simulink model "Linm_lin_1rob"  (Simulink 7.5)
settings: Solver=ode3  StartTime=0.0  StopTime=3  FixedStep=0.02  RelTol=1e-3
settings Model: Creator=FClaveau  LastModifiedBy=fclaveau
settings DebuggingCC: SaveWithParameterizedLinksMsg=none  MultiTaskCondExecSysMsg=none  StrictBusMsg=Warning
settings RTWCC: IncludeERTFirstTime=on

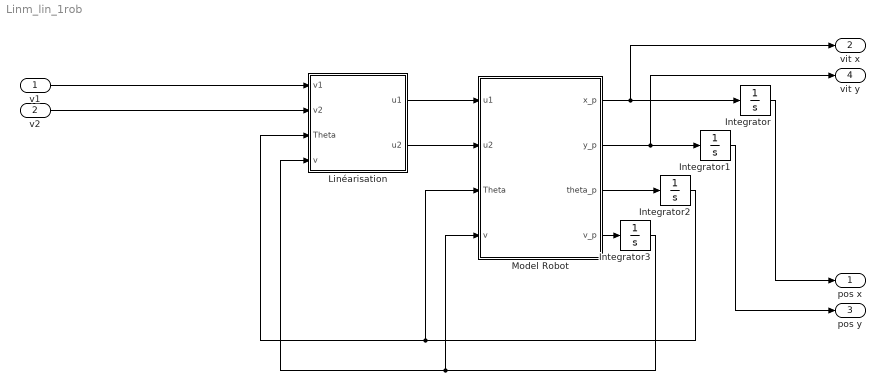
== system Linm_lin_1rob ==
  v1 : Inport
  v2 : Inport  Port=2
  Integrator : Integrator
  Integrator1 : Integrator
  Integrator2 : Integrator  InitialCondition=1
  Integrator3 : Integrator  InitialCondition=2
  Linéarisation : Subsystem
  Model Robot : Subsystem
  pos x : Outport
  vit x : Outport  Port=2
  pos y : Outport  Port=3
  vit y : Outport  Port=4
  wires:
  Model Robot/1(x_p) -> Integrator/1, vit x/1
  Model Robot/2(y_p) -> Integrator1/1, vit y/1
  Model Robot/3(theta_p) -> Integrator2/1
  Model Robot/4(v_p) -> Integrator3/1
  Integrator2/1 -> Model Robot/3(Theta), Linéarisation/3(Theta)
  Integrator3/1 -> Model Robot/4(v), Linéarisation/4(v)
  v2/1 -> Linéarisation/2(v2)
  Integrator/1 -> pos x/1
  Integrator1/1 -> pos y/1
  Linéarisation/1(u1) -> Model Robot/1(u1)
  Linéarisation/2(u2) -> Model Robot/2(u2)
  v1/1 -> Linéarisation/1(v1)

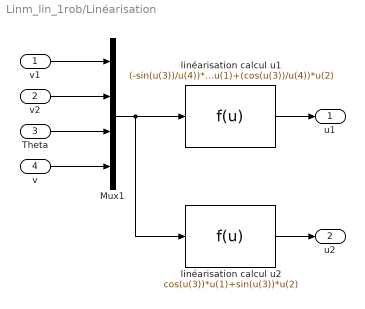
== system Linm_lin_1rob/Linéarisation ==
  v1 : Inport
  v2 : Inport  Port=2
  Theta : Inport  Port=3
  v : Inport  Port=4
  Mux1 : Mux
  linéarisation calcul u1 : Fcn  Expr=(-sin(u(3))/u(4))*u(1)+(cos(u(3))/u(4))*u(2)
  linéarisation calcul u2 : Fcn  Expr=cos(u(3))*u(1)+sin(u(3))*u(2)
  u1 : Outport
  u2 : Outport  Port=2
  wires:
  v1/1 -> Mux1/1
  v2/1 -> Mux1/2
  Theta/1 -> Mux1/3
  v/1 -> Mux1/4
  Mux1/1 -> linéarisation calcul u1/1, linéarisation calcul u2/1
  linéarisation calcul u2/1 -> u2/1
  linéarisation calcul u1/1 -> u1/1

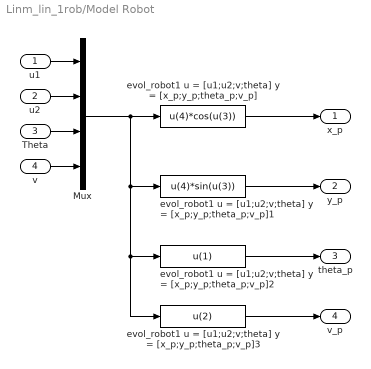
== system Linm_lin_1rob/Model Robot ==
  u1 : Inport
  u2 : Inport  Port=2
  Theta : Inport  Port=3
  v : Inport  Port=4
  Mux : Mux
  evol_robot1 u = [u1;u2;v;theta] y = [x_p;y_p;theta_p;v_p] : Fcn  Expr=u(4)*cos(u(3))
  evol_robot1 u = [u1;u2;v;theta] y = [x_p;y_p;theta_p;v_p]1 : Fcn  Expr=u(4)*sin(u(3))
  evol_robot1 u = [u1;u2;v;theta] y = [x_p;y_p;theta_p;v_p]2 : Fcn  Expr=u(1)
  evol_robot1 u = [u1;u2;v;theta] y = [x_p;y_p;theta_p;v_p]3 : Fcn  Expr=u(2)
  x_p : Outport
  y_p : Outport  Port=2
  theta_p : Outport  Port=3
  v_p : Outport  Port=4
  wires:
  evol_robot1 u = [u1;u2;v;theta] y = [x_p;y_p;theta_p;v_p]/1 -> x_p/1
  Mux/1 -> evol_robot1 u = [u1;u2;v;theta] y = [x_p;y_p;theta_p;v_p]/1, evol_robot1 u = [u1;u2;v;theta] y = [x_p;y_p;theta_p;v_p]1/1, evol_robot1 u = [u1;u2;v;theta] y = [x_p;y_p;theta_p;v_p]2/1, evol_robot1 u = [u1;u2;v;theta] y = [x_p;y_p;theta_p;v_p]3/1
  u1/1 -> Mux/1
  u2/1 -> Mux/2
  Theta/1 -> Mux/3
  v/1 -> Mux/4
  evol_robot1 u = [u1;u2;v;theta] y = [x_p;y_p;theta_p;v_p]1/1 -> y_p/1
  evol_robot1 u = [u1;u2;v;theta] y = [x_p;y_p;theta_p;v_p]2/1 -> theta_p/1
  evol_robot1 u = [u1;u2;v;theta] y = [x_p;y_p;theta_p;v_p]3/1 -> v_p/1
